simulink model "PLUTO_Rx"  (R2019a)
settings: Solver=FixedStepDiscrete  StartTime=0.0  StopTime=60  RelTol=1e-3
StartFcn:
  | tc = clock; %当前时间
  | time_str = sprintf('%d%02d%02d_%02d%02d%02d', tc(1),tc(2),tc(3),tc(4),tc(5),floor(tc(6)));
StopFcn:
  | system(['ren PLUTO_data.dat PLUTO_',time_str,'.dat'])
  | clearvars tc time_str
undefined symbols (not defined in the file or in its folder): Fs, ip, usb
libraries: plutoradiolib x1, dspsnks4 x1, simulink x1
settings Model: ModifiedComment=longt -- Fri Jul 26 10:36:19 2019 -- Version 1.25  Creator=longt  LastModifiedBy=longt
settings DataIOCC: SaveOutput=off  SignalLogging=off  DSMLogging=off  SaveTime=off  ReturnWorkspaceOutputs=off

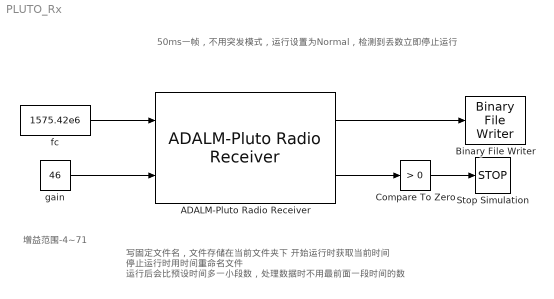
== system PLUTO_Rx ==
  note: 写固定文件名，文件存储在当前文件夹下
      | 开始运行时获取当前时间
      | 停止运行时用时间重命名文件
      | 运行后会比预设时间多一小段数，处理数据时不用最前面一段时间的数
  note: 增益范围-4~71
  note: 50ms一帧，不用突发模式，运行设置为Normal，检测到丢数立即停止运行
  ADALM-Pluto Radio Receiver : plutoradiolib/ADALM-Pluto Radio Receiver  RadioID=usb:0  uri=ip:10.0.0.200  CenterFrequencySource=Input Port  CenterFrequency=2.4e9  GainSource=AGC Slow Attack  GainSourceBlock=Input Port  Gain=10  ChannelMapping=1  BasebandSampleRate=4e6  OutputDataType=int16  SamplesPerFrame=2e5  OverflowOutputPort=on  EnableBurstMode=off  NumFramesInBurst=40  ShowAdvancedProperties=off  UseCustomFilter=off  filtPathRates=[737280000 11520000 3840000 1920000 960000 240000]  filtCoefficients=[-192 82 85 -215 228 -102 -110 290 -318 145 160 -426 471 -215 -238 633 -697 318 349 -923 1009 -457 -498 1309 -1423 640 693 -1812 1959 -876 -945 2458 -2647 1180 1268 -3290 3534 -1572 -1688 4375 -4698 2091 2247 -5836 6284 -2807 -3031 7918 -8588 3870 4225 -11182 12324 -5662 -6330 17255 -19735 9507 11312 -33568 43355 -25227 -42139 305542 305542 -42139 -25227 43355 -33568 11312 9507 -19735 17255 -6330 -5662 12324 -11182 4225 3870 -8588 7918 -3031 -2807 6284 -5836 2247 2091 -4698 4375 -1688 -1572 3534 -3290 1268 1180 -2647 2458 -945 -876 1959 -1812 693 640 -1423 1309 -498 -457 1009 -923 349 318 -697 633 -238 -215 471 -426 160 145 -318 290 -110 -102 228 -215 85 82 -192]  filtCoefficientSize=128  filtDecimInterpFactor=4  filtGain=-12  filtRFBandwidth=18000000  filterConfigStruct=struct()  EnableQuadratureCorrection=on  EnableRFDCCorrection=on  EnableBasebandDCCorrection=on  FrequencyCorrection=0  OverrideSampleTime=off  SampleTime=0.02  DataTimeout=Inf  ENSMPinControlMode=None  BISTLoopbackMode=Disabled  BISTToneInject=Disabled  BISTSignalGen=PRBS  BISTToneFreq=Fs/32  BISTToneLevel=0
      settings: SourceProductName=Communications Toolbox Support Package for Analog Devices ADALM-Pluto Radio  SourceProductBaseCode=PLUTO
  Binary File Writer : dspsnks4/Binary File Writer  Filename=PLUTO_data.dat  HeaderStructure=struct([])  SimulateUsing=Interpreted execution
      settings: SourceProductName=DSP System Toolbox  SourceProductBaseCode=DS
  Compare To Zero : simulink/Logic and Bit Operations/Compare To Zero  relop=>  OutDataTypeStr=boolean
  Stop Simulation : Stop
  fc : Constant  Value=1575.42e6  OutMin=325e6  OutMax=3800e6
  gain : Constant  Value=46  OutMin=-4  OutMax=71
  wires:
  fc/1 -> ADALM-Pluto Radio Receiver/1
  gain/1 -> ADALM-Pluto Radio Receiver/2
  ADALM-Pluto Radio Receiver/1 -> Binary File Writer/1
  ADALM-Pluto Radio Receiver/2 -> Compare To Zero/1
  Compare To Zero/1 -> Stop Simulation/1
